simulink model "error"  (R2023b)
settings: Solver=VariableStepAuto  StartTime=0.0  StopTime=30  RelTol=1e-3
values from neighbouring files (symbols this model uses):
  A = sys_d.A    [error_dynamic.m]
  B = sys_d.B    [error_dynamic.m]
  C = sys_d.C    [error_dynamic.m]
  E = Es * Wr    [error_dynamic.m]
  K = place(A,B,p0)    [error_dynamic.m]
  Ts = 0.25    [error_dynamic.m]
  x0 = [0.8;0.2;-0.6;0]    [error_dynamic.m]
libraries: slpidlib x1
settings Model: Creator=Fan Xiuqi  LastModifiedBy=Fan Xiuqi

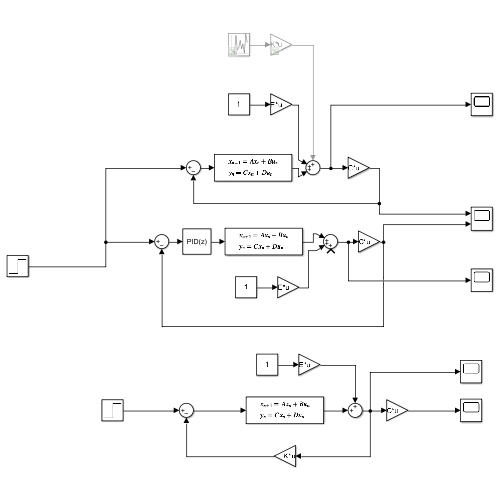
[thumbnail: Simulink's stored preview of the top-level diagram]
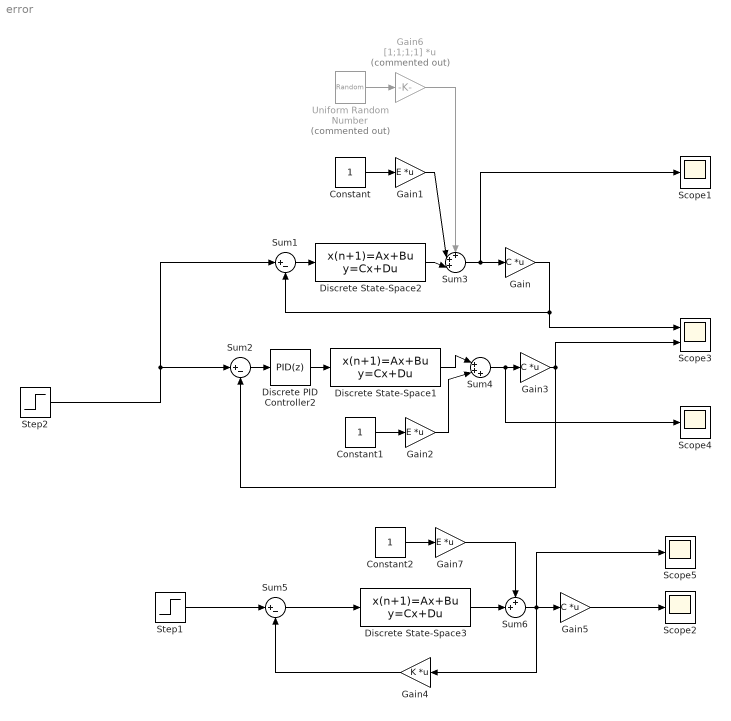
== system error ==
  Constant : Constant  SampleTime=Ts
  Constant1 : Constant  SampleTime=Ts
  Constant2 : Constant  SampleTime=Ts
  Discrete PID Controller2 : slpidlib/PID Controller  Controller=PID  Form=Parallel  TimeDomain=Discrete-time  UseExternalTs=off  SampleTime=-1  IntegratorMethod=Forward Euler  FilterMethod=Forward Euler  ControllerParametersSource=internal  P=0.4  I=0.06  UseKiTs=off  D=0.1  N=100  UseFilter=off  TunerSelectOption=Transfer Function Based (PID Tuner App)  InitialConditionSource=internal  InitialConditionForIntegrator=0  InitialConditionForFilter=0  DifferentiatorICPrevScaledInput=0  ExternalReset=none  TrackingMode=off  Kt=1  LimitOutput=off  SatLimitsSource=internal  UpperSaturationLimit=inf  LowerSaturationLimit=-inf  LinearizeAsGain=off  AntiWindupMode=none  Kb=1  LimitIntegrator=off  UpperIntegratorSaturationLimit=inf  LowerIntegratorSaturationLimit=-inf  POutMin=[]  POutMax=[]  IOutMin=[]  IOutMax=[]  DOutMin=[]  DOutMax=[]  NOutMin=[]  NOutMax=[]  SumOutMin=[]  SumOutMax=[]  SaturationOutMin=[]  SaturationOutMax=[]  PParamMin=[]  PParamMax=[]  IParamMin=[]  IParamMax=[]  DParamMin=[]  DParamMax=[]  NParamMin=[]  NParamMax=[]  KbParamMin=[]  KbParamMax=[]  KtParamMin=[]  KtParamMax=[]  KbOutMin=[]  KbOutMax=[]  KtOutMin=[]  KtOutMax=[]  IntegratorOutMin=[]  IntegratorOutMax=[]  FilterOutMin=[]  FilterOutMax=[]  SumI1OutMin=[]  SumI1OutMax=[]  SumI2OutMin=[]  SumI2OutMax=[]  SumI3OutMin=[]  SumI3OutMax=[]  SumI4OutMin=[]  SumI4OutMax=[]  SumDOutMin=[]  SumDOutMax=[]  DifferentiatorOutMin=[]  DifferentiatorOutMax=[]  FilterDiffOutCoefMin=[]  FilterDiffOutCoefMax=[]  ReciprocalOutMin=[]  ReciprocalOutMax=[]  SumDenOutMin=[]  SumDenOutMax=[]  SumNumOutMin=[]  SumNumOutMax=[]  DivideOutMin=[]  DivideOutMax=[]  UdiffTsProdOutMin=[]  UdiffTsProdOutMax=[]  NTsProdOutMin=[]  NTsProdOutMax=[]  UintegralTsProdOutMin=[]  UintegralTsProdOutMax=[]  UngainTsProdOutMin=[]  UngainTsProdOutMax=[]  ClampingZeroOutDataTypeStr=Inherit: Inherit via back propagation  ClampingZeroOutMin=[]  ClampingZeroOutMax=[]  FilterDenConstantOutDataTypeStr=Inherit: Inherit via back propagation  FilterDenConstantOutMin=[]  FilterDenConstantOutMax=[]  PCopyOutDataTypeStr=Inherit: Inherit via back propagation  PCopyOutMin=[]  PCopyOutMax=[]  NCopyOutDataTypeStr=Inherit: Inherit via back propagation  NCopyOutMin=[]  NCopyOutMax=[]  IntegratorContinuousStateAttributes=''  IntegratorStateMustResolveToSignalObject=off  IntegratorRTWStateStorageClass=Auto  FilterContinuousStateAttributes=''  FilterStateMustResolveToSignalObject=off  FilterRTWStateStorageClass=Auto  ParallelPVariant=InternalParameters  IdealPVariant=Disabled  IVariant=InternalParameters  DVariant=InternalParameters  IntegratorVariant=Discrete  SatVariant=Disabled  AWVariant=Passthrough  PCopyVariant=Disabled  TRVariant=Disabled  FdbkBlocksVariant=Forward  IdealPFdbkVariant=Disabled  SatFdbkVariant=Disabled  DerivativeFilterVariant=Differentiator  NVariant=Passthrough  NCopyVariant=Disabled_SignalSpec  FilterICVariant=InternalICsDifferentiator  IntegratorICVariant=InternalICs  ExternalResetVariant=Disabled  TRSumVariant=Passthrough  SumFdbkVariant=Disabled  SumVariant=Sum_PID  TsampFilterVariant=InternalTs  TsampNgainVariant=Passthrough  TsampIntegralVariant=Disabled_SignalSpec  ExternalSaturationOutDataTypeStr=Inherit: Same as second input
      settings: LibrarySourceBlock=simulink/Discrete/Discrete PID Controller
  Discrete State-Space1 : DiscreteStateSpace  A=A  B=B  C=eye(4)  D=zeros(4,1)  InitialCondition=x0  SampleTime=Ts
  Discrete State-Space2 : DiscreteStateSpace  A=A  B=B  C=eye(4)  D=zeros(4,1)  InitialCondition=x0  SampleTime=Ts
  Discrete State-Space3 : DiscreteStateSpace  A=A  B=B  C=eye(4)  D=zeros(4,1)  InitialCondition=x0  SampleTime=Ts
  Gain : Gain  Gain=C  Multiplication=Matrix(K*u)
  Gain1 : Gain  Gain=E  Multiplication=Matrix(K*u)
  Gain2 : Gain  Gain=E  Multiplication=Matrix(K*u)
  Gain3 : Gain  Gain=C  Multiplication=Matrix(K*u)
  Gain4 : Gain  Gain=K  Multiplication=Matrix(K*u)
  Gain5 : Gain  Gain=C  Multiplication=Matrix(K*u)
  Gain6 : Gain  Commented=on  Gain=[1;1;1;1]  Multiplication=Matrix(K*u)
  Gain7 : Gain  Gain=E  Multiplication=Matrix(K*u)
  Scope{1..2,4..5} (4 alike) : Scope
  Scope3 : Scope  NumInputPorts=2
  Step1 : Step  SampleTime=Ts
  Step2 : Step  SampleTime=Ts
  Sum1 : Sum  Inputs=|+-
  Sum2 : Sum  Inputs=|+-
  Sum3 : Sum  Inputs=+++|
  Sum4 : Sum  Inputs=|+++
  Sum5 : Sum  Inputs=|+-
  Sum6 : Sum  Inputs=++|
  Uniform Random Number : UniformRandomNumber  Commented=on  Minimum=-0.1  Maximum=0.1  SampleTime=Ts
  wires:
  Sum1/1 -> Discrete State-Space2/1
  Gain/1 -> Scope3/1, Sum1/2
  Sum3/1 -> Scope1/1, Gain/1
  Constant/1 -> Gain1/1
  Constant1/1 -> Gain2/1
  Discrete State-Space1/1 -> Sum4/1
  Sum4/1 -> Scope4/1, Gain3/1
  Gain2/1 -> Sum4/2
  Gain3/1 -> Sum2/2, Scope3/2
  Sum2/1 -> Discrete PID Controller2/1
  Discrete PID Controller2/1 -> Discrete State-Space1/1
  Step2/1 -> Sum1/1, Sum2/1
  Sum5/1 -> Discrete State-Space3/1
  Step1/1 -> Sum5/1
  Gain4/1 -> Sum5/2
  Gain5/1 -> Scope2/1
  Uniform Random Number/1 -> Gain6/1
  Discrete State-Space2/1 -> Sum3/3
  Gain1/1 -> Sum3/2
  Gain6/1 -> Sum3/1
  Discrete State-Space3/1 -> Sum6/2
  Sum6/1 -> Scope5/1, Gain4/1, Gain5/1
  Constant2/1 -> Gain7/1
  Gain7/1 -> Sum6/1
